simulink model "circuit_hidraulic_R2022b"  (R2024b)
settings: Solver=FixedStepAuto  StartTime=0.0  StopTime=Tfin  FixedStep=Ts  RelTol=1e-3
values from neighbouring files (symbols this model uses):
  a1 = 2*c2*c1    (= 1.76)    [ILBAN_Alessandro_setup_circuit_hidraulic_chirp.m]
  a2 = c1    (= 0.55)    [ILBAN_Alessandro_setup_circuit_hidraulic_chirp.m]
  Ain = 1.4    [ILBAN_Alessandro_setup_circuit_hidraulic_chirp.m]
  b0 = (1.2+m+n)/5.5    (= 3.49090909091)    [ILBAN_Alessandro_setup_circuit_hidraulic_chirp.m]
  Tfin = 30*c2/c1*10    (= 872.727272727)    [ILBAN_Alessandro_setup_circuit_hidraulic_chirp.m]
  Ts = 10*c2/c1/1e4*1.5    (= 0.00436363636364)    [ILBAN_Alessandro_setup_circuit_hidraulic_chirp.m]
  u_op_region = (m/2+n/5)/2    (= 2.25)    [ILBAN_Alessandro_setup_circuit_hidraulic_chirp.m]
  umax = gain    (= 10)    [ILBAN_Alessandro_setup_circuit_hidraulic_chirp.m]
  umin = 0    [ILBAN_Alessandro_setup_circuit_hidraulic_chirp.m]
  whtn_pow_in = 1e-6*5*(((m-1)*8+n/2)/5)/2*6/8    (= 8.8125e-06)    [ILBAN_Alessandro_setup_circuit_hidraulic_chirp.m]
  whtn_pow_out = 1e-5*5*(((m-1)*25+n/2)/5)*6/80*(0.5+0.3*(m-2))    (= 3.45e-05)    [ILBAN_Alessandro_setup_circuit_hidraulic_chirp.m]
  whtn_seed_in = 23341+m+2*n    (= 23374)    [ILBAN_Alessandro_setup_circuit_hidraulic_chirp.m]
  whtn_seed_out = 23342-m-2*n    (= 23309)    [ILBAN_Alessandro_setup_circuit_hidraulic_chirp.m]
  whtn_Ts_in = Ts*3    (= 0.0130909090909)    [ILBAN_Alessandro_setup_circuit_hidraulic_chirp.m]
  whtn_Ts_out = Ts*5    (= 0.0218181818182)    [ILBAN_Alessandro_setup_circuit_hidraulic_chirp.m]
  x0_slx = [2*(m/2+rand(1)*m/5); m*(n/20+rand(1)*n/100)]    [ILBAN_Alessandro_setup_circuit_hidraulic_chirp.m]
  ymax = b0*gain/1.5    (= 23.2727272727)    [ILBAN_Alessandro_setup_circuit_hidraulic_chirp.m]
  ymin = 0    [ILBAN_Alessandro_setup_circuit_hidraulic_chirp.m]
libraries: simulink x3
settings Model: Creator=mircea  LastModifiedBy=anter

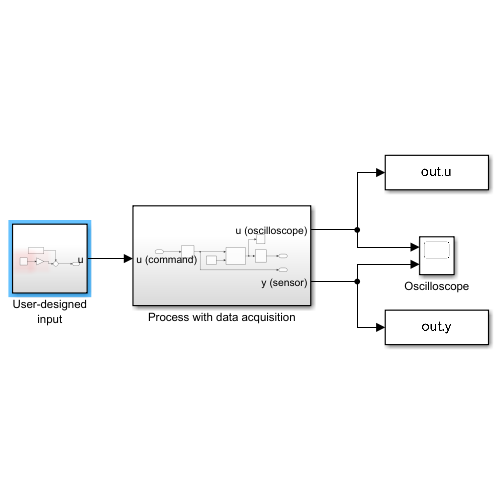
[thumbnail: Simulink's stored preview of the top-level diagram]
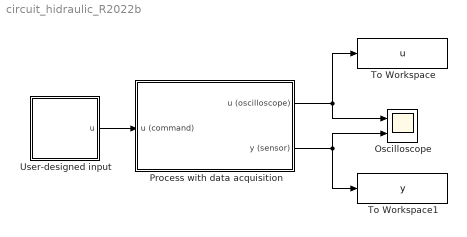
== system circuit_hidraulic_R2022b ==
  Oscilloscope : Scope  NumInputPorts=2
  Process with data acquisition : Subsystem
  To Workspace : ToWorkspace  VariableName=u  SampleTime=Ts
  To Workspace1 : ToWorkspace  VariableName=y  SampleTime=Ts
  User-designed input : Subsystem
  wires:
  Process with data acquisition/1(u (oscilloscope)) -> Oscilloscope/1, To Workspace/1
  Process with data acquisition/2(y (sensor)) -> Oscilloscope/2, To Workspace1/1
  User-designed input/1(u) -> Process with data acquisition/1(u (command))

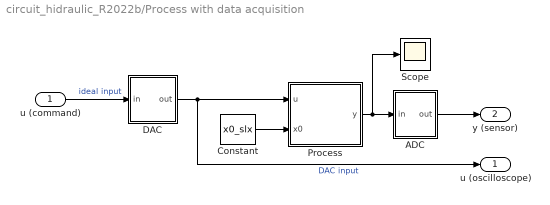
== system circuit_hidraulic_R2022b/Process with data acquisition ==
  u (command) : Inport
  ADC : Subsystem
  Constant : Constant  Value=x0_slx
  DAC : Subsystem
  Process : Subsystem
  Scope : Scope
  u (oscilloscope) : Outport
  y (sensor) : Outport  Port=2
  wires:
  Constant/1 -> Process/2(x0)
  u (command)/1 -> DAC/1(in)  "ideal input"
  Process/1(y) -> Scope/1, ADC/1(in)
  ADC/1(out) -> y (sensor)/1
  DAC/1(out) -> Process/1(u), u (oscilloscope)/1  "DAC input"

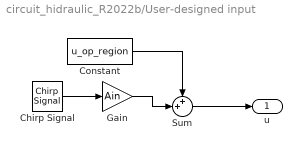
== system circuit_hidraulic_R2022b/User-designed input ==
  Chirp Signal : simulink/Sources/Chirp Signal  f1=fmin  T=Tfin  f2=fmax
  Constant : Constant  Value=u_op_region
  Gain : Gain  Gain=Ain
  Sum : Sum  Inputs=++|
  u : Outport
  wires:
  Constant/1 -> Sum/1
  Sum/1 -> u/1
  Chirp Signal/1 -> Gain/1
  Gain/1 -> Sum/2

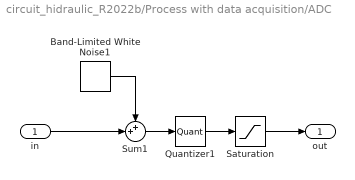
== system circuit_hidraulic_R2022b/Process with data acquisition/ADC ==
  in : Inport
  Band-Limited White Noise1 : simulink/Sources/Band-Limited White Noise  Cov=[whtn_pow_out]  Ts=whtn_Ts_out  seed=[whtn_seed_out]
  Quantizer1 : Quantizer  QuantizationInterval=q_out
  Saturation : Saturate  UpperLimit=ymax  LowerLimit=ymin
  Sum1 : Sum  Inputs=++|
  out : Outport
  wires:
  Quantizer1/1 -> Saturation/1
  Sum1/1 -> Quantizer1/1
  in/1 -> Sum1/2
  Band-Limited White Noise1/1 -> Sum1/1
  Saturation/1 -> out/1

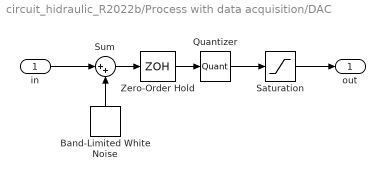
== system circuit_hidraulic_R2022b/Process with data acquisition/DAC ==
  in : Inport
  Band-Limited White Noise : simulink/Sources/Band-Limited White Noise  Cov=[whtn_pow_in]  Ts=whtn_Ts_in  seed=[whtn_seed_in]
  Quantizer : Quantizer  QuantizationInterval=q_in
  Saturation : Saturate  UpperLimit=umax  LowerLimit=umin
  Sum : Sum  Inputs=|++
  Zero-Order Hold : ZeroOrderHold  SampleTime=-1
  out : Outport
  wires:
  Quantizer/1 -> Saturation/1
  Sum/1 -> Zero-Order Hold/1
  in/1 -> Sum/1
  Band-Limited White Noise/1 -> Sum/2
  Zero-Order Hold/1 -> Quantizer/1
  Saturation/1 -> out/1

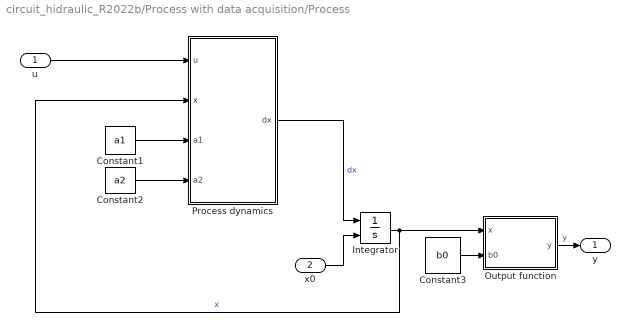
== system circuit_hidraulic_R2022b/Process with data acquisition/Process ==
  u : Inport
  x0 : Inport  Port=2
  Constant1 : Constant  Value=a1
  Constant2 : Constant  Value=a2
  Constant3 : Constant  Value=b0
  Integrator : Integrator  InitialConditionSource=external
  Output function : MATLAB Function  TreatAsAtomicUnit=on
  Process dynamics : MATLAB Function  TreatAsAtomicUnit=on
  y : Outport
  wires:
  u/1 -> Process dynamics/1(u)
  Process dynamics/1(dx) -> Integrator/1  "dx"
  Integrator/1 -> Output function/1(x), Process dynamics/2(x)  "x"
  Output function/1(y) -> y/1  "y"
  x0/1 -> Integrator/2
  Constant2/1 -> Process dynamics/4(a2)
  Constant1/1 -> Process dynamics/3(a1)
  Constant3/1 -> Output function/2(b0)

== matlab function circuit_hidraulic_R2022b/Process with data acquisition/Process/Process dynamics ==
  data: u input; dx output; x input; a1 input; a2 input
function dx = fcn(u,x,a1,a2)
dx = [-a1*x(1) - a2*x(2) + a2*u; a2*x(1)];

== matlab function circuit_hidraulic_R2022b/Process with data acquisition/Process/Output function ==
  data: y output; x input; b0 input
function y = fcn(x,b0)

y = b0*x(2);

end
